simulink model "simulate_controller"  (R2024a)
settings: Solver=VariableStepAuto  StartTime=-120  StopTime=360  MaxStep=0.1  RelTol=1e-3
values from neighbouring files (symbols this model uses):
  lower_lim_I = K_lims(1)    [Figure_4_simulations.m]    (also in generate_controllers.m)
  upper_lim_I = K_lims(2)    [Figure_4_simulations.m]    (also in generate_controllers.m)
libraries: cstblocks x4, slpidlib x1
settings Model: Creator=Denis  LastModifiedBy=denisroutkevitch
settings OptimizationCC: ReuseModelBlockBuffer=off
settings RTWCC: GPUComputeCapability=3.5

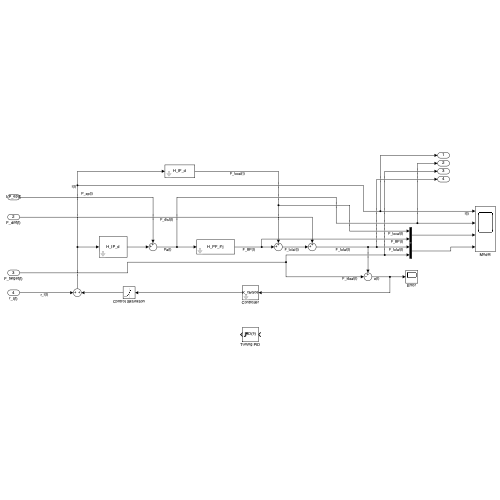
[thumbnail: Simulink's stored preview of the top-level diagram]
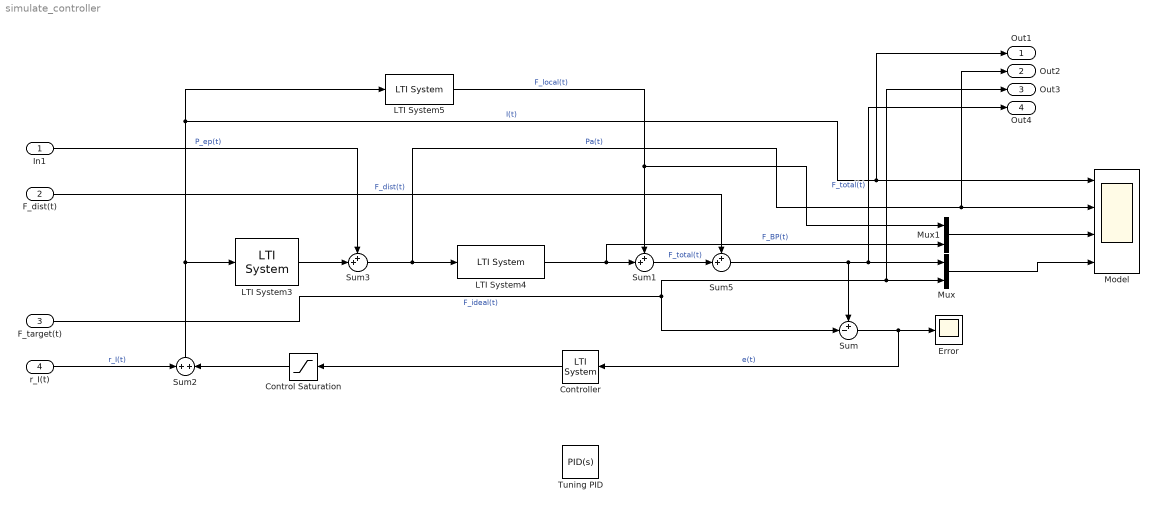
== system simulate_controller ==
  In1 : Inport
  "F_dist(t) " : Inport  Port=2
  F_target(t) : Inport  Port=3
  r_I(t) : Inport  Port=4
  Control Saturation : Saturate  UpperLimit=upper_lim_I  LowerLimit=lower_lim_I
  Controller : cstblocks/LTI System  sys=K_choice  IC=[]  PadeOrder=0
  Error : Scope
  LTI System3 : cstblocks/LTI System  sys=H_IP_d  IC=[]  PadeOrder=0
  LTI System4 : cstblocks/LTI System  sys=H_PF_inj  IC=[]  PadeOrder=0
  LTI System5 : cstblocks/LTI System  sys=H_IF_d  IC=[]  PadeOrder=0
  Model : Scope  NumInputPorts=4
  Mux : Mux  Inputs=2
  Mux1 : Mux  Inputs=2
  Sum : Sum  Inputs=+-|
  Sum1 : Sum  Inputs=++|
  Sum2 : Sum  Inputs=+|+
  Sum3 : Sum  Inputs=++|
  Sum5 : Sum  Inputs=++|
  Tuning PID : slpidlib/PID Controller  Controller=PID  Form=Parallel  TimeDomain=Continuous-time  UseExternalTs=off  SampleTime=-1  IntegratorMethod=Forward Euler  FilterMethod=Forward Euler  ControllerParametersSource=internal  P=-0.000571429039548576  I=-6.4935874741923e-06  UseKiTs=off  D=0.0150267772530542  UseExternalDerivativeSource=off  N=0.0251494937579228  UseFilter=on  TunerSelectOption=Transfer Function Based (PID Tuner App)  InitialConditionSource=internal  InitialConditionForIntegrator=0  InitialConditionForFilter=0  DifferentiatorICPrevScaledInput=0  ExternalReset=none  TrackingMode=off  Kt=1  LimitOutput=on  SatLimitsSource=internal  UpperSaturationLimit=inf  LowerSaturationLimit=-inf  LinearizeAsGain=on  AntiWindupMode=none  Kb=1  LimitIntegrator=off  UpperIntegratorSaturationLimit=inf  LowerIntegratorSaturationLimit=-inf  POutMin=[]  POutMax=[]  IOutMin=[]  IOutMax=[]  DOutMin=[]  DOutMax=[]  NOutMin=[]  NOutMax=[]  SumOutMin=[]  SumOutMax=[]  SaturationOutMin=[]  SaturationOutMax=[]  PParamMin=[]  PParamMax=[]  IParamMin=[]  IParamMax=[]  DParamMin=[]  DParamMax=[]  NParamMin=[]  NParamMax=[]  KbParamMin=[]  KbParamMax=[]  KtParamMin=[]  KtParamMax=[]  KbOutMin=[]  KbOutMax=[]  KtOutMin=[]  KtOutMax=[]  IntegratorOutMin=[]  IntegratorOutMax=[]  FilterOutMin=[]  FilterOutMax=[]  SumI1OutMin=[]  SumI1OutMax=[]  SumI2OutMin=[]  SumI2OutMax=[]  SumI3OutMin=[]  SumI3OutMax=[]  SumI4OutMin=[]  SumI4OutMax=[]  SumDOutMin=[]  SumDOutMax=[]  DifferentiatorOutMin=[]  DifferentiatorOutMax=[]  FilterDiffOutCoefMin=[]  FilterDiffOutCoefMax=[]  ReciprocalOutMin=[]  ReciprocalOutMax=[]  SumDenOutMin=[]  SumDenOutMax=[]  SumNumOutMin=[]  SumNumOutMax=[]  DivideOutMin=[]  DivideOutMax=[]  UdiffTsProdOutMin=[]  UdiffTsProdOutMax=[]  NTsProdOutMin=[]  NTsProdOutMax=[]  UintegralTsProdOutMin=[]  UintegralTsProdOutMax=[]  UngainTsProdOutMin=[]  UngainTsProdOutMax=[]  ClampingZeroOutDataTypeStr=Inherit: Inherit via back propagation  ClampingZeroOutMin=[]  ClampingZeroOutMax=[]  FilterDenConstantOutDataTypeStr=Inherit: Inherit via back propagation  FilterDenConstantOutMin=[]  FilterDenConstantOutMax=[]  PCopyOutDataTypeStr=Inherit: Inherit via back propagation  PCopyOutMin=[]  PCopyOutMax=[]  NCopyOutDataTypeStr=Inherit: Inherit via back propagation  NCopyOutMin=[]  NCopyOutMax=[]  IntegratorContinuousStateAttributes=''  IntegratorStateMustResolveToSignalObject=off  IntegratorRTWStateStorageClass=Auto  FilterContinuousStateAttributes=''  FilterStateMustResolveToSignalObject=off  FilterRTWStateStorageClass=Auto  ParallelPVariant=InternalParameters  IdealPVariant=Disabled  IVariant=InternalParameters  DVariant=InternalParameters  IntegratorVariant=Continuous  SatVariant=Enabled  AWVariant=Passthrough  PCopyVariant=Disabled  TRVariant=Disabled  FdbkBlocksVariant=Forward  IdealPFdbkVariant=Disabled  SatFdbkVariant=Disabled  DerivativeFilterVariant=ContFilter  NVariant=InternalParameters  NCopyVariant=Disabled  FilterICVariant=InternalICsFilter  IntegratorICVariant=InternalICs  ExternalResetVariant=Disabled  TRSumVariant=Passthrough  SumFdbkVariant=Disabled  SumVariant=Sum_PID  TsampFilterVariant=InternalTs  TsampNgainVariant=Passthrough  TsampIntegralVariant=Disabled_SignalSpec  ExternalSaturationOutDataTypeStr=Inherit: Same as second input  DerivativeSourceVariant=ErrorSignal
  Out1 : Outport
  Out2 : Outport  Port=2
  Out3 : Outport  Port=3
  Out4 : Outport  Port=4
  wires:
  Sum/1 -> Controller/1, Error/1  "e(t)"
  r_I(t)/1 -> Sum2/1  "r_I(t)"
  LTI System4/1 -> Mux1/2, Sum1/2  "F_BP(t)"
  LTI System5/1 -> Sum1/1, Mux1/1  "F_local(t)"
  Sum3/1 -> Out2/1, Model/2, LTI System4/1  "Pa(t)"
  LTI System3/1 -> Sum3/2
  Sum5/1 -> Sum/1, Out4/1, Mux/1  "F_total(t)"
  In1/1 -> Sum3/1  "P_ep(t)"
  Sum2/1 -> LTI System5/1, Out1/1, Model/1, LTI System3/1  "I(t)"
  F_target(t)/1 -> Sum/2, Out3/1, Mux/2  "F_ideal(t)"
  Mux/1 -> Model/4
  Mux1/1 -> Model/3
  Control Saturation/1 -> Sum2/2
  "F_dist(t) "/1 -> Sum5/1  "F_dist(t)"
  Sum1/1 -> Sum5/2  "F_total(t)"
  Controller/1 -> Control Saturation/1
